simulink library "halout"  (R2021b)
settings: Solver=VariableStepAuto  StartTime=0.0  StopTime=10.0  RelTol=1e-3
undefined symbols (not defined in the file): C_TASK_5MS_S, FALSE, KHAL_CAN1TxReq_flg, KHAL_CAN2TxReq_flg, KHAL_CAN3FD3VCU1toNIDECTxReq_flg, KHAL_CAN3FD3VCU1TxReq_flg, KHAL_CAN3FD3VCU2E2E_flg, KHAL_CAN3FD3VCU2toNIDECE2E_flg, KHAL_CAN3FD3VCU2toNIDECTxReq_flg, KHAL_CAN3FD3VCU2TxReq_flg, KHAL_CAN3TxReq_flg, KHAL_CAN4FD4CE1000E2E_flg, KHAL_CAN4FD4CE1000TxReq_flg, KHAL_CAN4TxReq_flg, KHAL_CAN5TxReq_flg, KHAL_CAN7TxReq_flg, ONE_INT, TRUE, ZERO_INT
libraries: FVT_lib x258, simulink x115
(part 2 of 17)

== system halout/HAL_OUT/CAN1/GW1_C1000_1_0x18E0FF21 ==
  BSCP_outputs : Inport  OutDataTypeStr=Bus: BSCP_outputs
  BOUTP_outputs : Inport  Port=2  OutDataTypeStr=Bus: BOUTP_outputs
  SeatBeltSwitch : Subsystem
  bus_creator : BusCreator  Inputs=1  OutDataTypeStr=Bus: DT_CAN1_SG_GW1_C1000_1  NonVirtualBus=on
  bus_selector : BusSelector  OutputSignals=VOUTP_SeatBeltSwitch_enum
  GW1_C1000_1 : Outport
  wires:
  BSCP_outputs/1 -> [BSCP_outputs]
  BOUTP_outputs/1 -> [BOUTP_outputs]
  [CAN1_SeatBeltSwitch] -> bus_creator/1  "CAN1_SeatBeltSwitch"
  bus_creator/1 -> GW1_C1000_1/1
  SeatBeltSwitch/1(CAN1_SeatBeltSwitch) -> [CAN1_SeatBeltSwitch]
  bus_selector/1 -> SeatBeltSwitch/1(SeatBeltSwitch)  "<VOUTP_SeatBeltSwitch_enum>"
  [BOUTP_outputs] -> bus_selector/1

== system halout/HAL_OUT/CAN1/GW1_C100_4_0x18FDA521 ==
  BSCP_outputs : Inport  OutDataTypeStr=Bus: BSCP_outputs
  BOUTP_outputs : Inport  Port=2  OutDataTypeStr=Bus: BOUTP_outputs
  OpenStatusOfDoor1 : Subsystem
  OpenStatusOfDoor2 : Subsystem
  bus_creator : BusCreator  Inputs=2  OutDataTypeStr=Bus: DT_CAN1_SG_GW1_C100_4  NonVirtualBus=on
  bus_selector : BusSelector  OutputSignals=VOUTP_OpenStatusOfDoor1_enum
  bus_selector1 : BusSelector  OutputSignals=VOUTP_OpenStatusOfDoor2_enum
  GW1_C100_4 : Outport
  wires:
  BSCP_outputs/1 -> [BSCP_outputs]
  BOUTP_outputs/1 -> [BOUTP_outputs]
  [CAN1_OpenStatusOfDoor1] -> bus_creator/1  "CAN1_OpenStatusOfDoor1"
  [CAN1_OpenStatusOfDoor2] -> bus_creator/2  "CAN1_OpenStatusOfDoor2"
  bus_creator/1 -> GW1_C100_4/1
  OpenStatusOfDoor1/1(CAN1_OpenStatusOfDoor1) -> [CAN1_OpenStatusOfDoor1]
  OpenStatusOfDoor2/1(CAN1_OpenStatusOfDoor2) -> [CAN1_OpenStatusOfDoor2]
  bus_selector/1 -> OpenStatusOfDoor1/1(OpenStatusOfDoor1)  "<VOUTP_OpenStatusOfDoor1_enum>"
  [BOUTP_outputs] -> bus_selector/1
  bus_selector1/1 -> OpenStatusOfDoor2/1(OpenStatusOfDoor2)  "<VOUTP_OpenStatusOfDoor2_enum>"
  [BOUTP_outputs] -> bus_selector1/1

== system halout/HAL_OUT/CAN1/VCU_PDU_Demand_1_0xCF101D0 ==
  BSCP_outputs : Inport  OutDataTypeStr=Bus: BSCP_outputs
  BOUTP_outputs : Inport  Port=2  OutDataTypeStr=Bus: BOUTP_outputs
  DCDCRlyEn : Subsystem
  EACRlyEn : Subsystem
  EHPSRlyEn : Subsystem
  Ground : Ground
  VCULife1 : Subsystem
  bus_creator : BusCreator  Inputs=4  OutDataTypeStr=Bus: DT_CAN1_SG_VCU_PDU_Demand_1  NonVirtualBus=on
  bus_selector : BusSelector  OutputSignals=VOUTP_DCDCRlyDem_enum
  bus_selector1 : BusSelector  OutputSignals=VOUTP_EACRlyDem_enum
  bus_selector2 : BusSelector  OutputSignals=VOUTP_EHPSRlyDem_enum
  VCU_PDU_Demand_1 : Outport
  wires:
  BSCP_outputs/1 -> [BSCP_outputs]
  BOUTP_outputs/1 -> [BOUTP_outputs]
  [CAN1_DCDCRlyEn] -> bus_creator/1  "CAN1_DCDCRlyEn"
  [CAN1_EACRlyEn] -> bus_creator/2  "CAN1_EACRlyEn"
  [CAN1_EHPSRlyEn] -> bus_creator/3  "CAN1_EHPSRlyEn"
  [CAN1_VCULife1] -> bus_creator/4  "CAN1_VCULife1"
  bus_creator/1 -> VCU_PDU_Demand_1/1
  DCDCRlyEn/1(CAN1_DCDCRlyEn) -> [CAN1_DCDCRlyEn]
  EACRlyEn/1(CAN1_EACRlyEn) -> [CAN1_EACRlyEn]
  EHPSRlyEn/1(CAN1_EHPSRlyEn) -> [CAN1_EHPSRlyEn]
  VCULife1/1(CAN1_VCULife1) -> [CAN1_VCULife1]
  bus_selector/1 -> DCDCRlyEn/1(DCDCRlyEn)  "<VOUTP_DCDCRlyDem_enum>"
  [BOUTP_outputs] -> bus_selector/1
  bus_selector1/1 -> EACRlyEn/1(EACRlyEn)  "<VOUTP_EACRlyDem_enum>"
  [BOUTP_outputs] -> bus_selector1/1
  bus_selector2/1 -> EHPSRlyEn/1(EHPSRlyEn)  "<VOUTP_EHPSRlyDem_enum>"
  [BOUTP_outputs] -> bus_selector2/1
  Ground/1 -> VCULife1/1(VCULife1)

== system halout/HAL_OUT/CAN2/FD2_C200_1_0x18F001EF ==
  BSCP_outputs : Inport  OutDataTypeStr=Bus: BSCP_outputs
  BOUTP_outputs : Inport  Port=2  OutDataTypeStr=Bus: BOUTP_outputs
  FDCCHACACPresWarnSta : Subsystem
  FDCCHACACTempWarnSta : Subsystem
  bus_creator : BusCreator  Inputs=2  OutDataTypeStr=Bus: DT_CAN2_SG_FD2_C200_1  NonVirtualBus=on
  bus_selector : BusSelector  OutputSignals=VOUTP_CACPresWarnSta_flg
  bus_selector1 : BusSelector  OutputSignals=VOUTP_CACTempWarnSta_flg
  FD2_C200_1 : Outport
  wires:
  BSCP_outputs/1 -> [BSCP_outputs]
  BOUTP_outputs/1 -> [BOUTP_outputs]
  [CAN2_FDC_CHA_CACPresWarn_Sta] -> bus_creator/1  "CAN2_FDC_CHA_CACPresWarn_Sta"
  [CAN2_FDC_CHA_CACTempWarn_Sta] -> bus_creator/2  "CAN2_FDC_CHA_CACTempWarn_Sta"
  bus_creator/1 -> FD2_C200_1/1
  FDCCHACACPresWarnSta/1(CAN2_FDC_CHA_CACPresWarn_Sta) -> [CAN2_FDC_CHA_CACPresWarn_Sta]
  FDCCHACACTempWarnSta/1(CAN2_FDC_CHA_CACTempWarn_Sta) -> [CAN2_FDC_CHA_CACTempWarn_Sta]
  bus_selector/1 -> FDCCHACACPresWarnSta/1(FDCCHACACPresWarnSta)  "<VOUTP_CACPresWarnSta_flg>"
  [BOUTP_outputs] -> bus_selector/1
  bus_selector1/1 -> FDCCHACACTempWarnSta/1(FDCCHACACTempWarnSta)  "<VOUTP_CACTempWarnSta_flg>"
  [BOUTP_outputs] -> bus_selector1/1

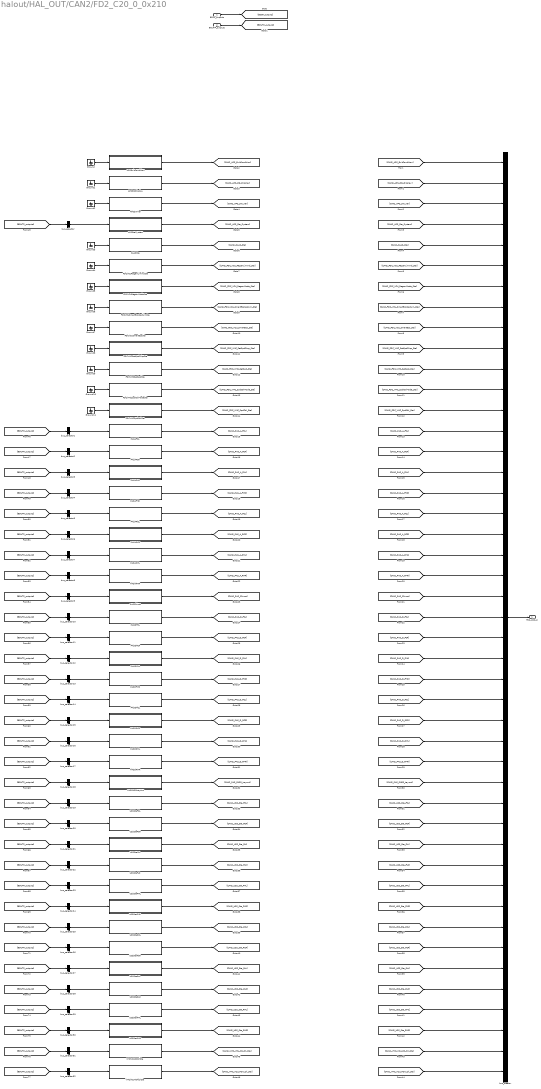
== system halout/HAL_OUT/CAN2/FD2_C20_0_0x210 ==
  BSCP_outputs : Inport  OutDataTypeStr=Bus: BSCP_outputs
  BOUTP_outputs : Inport  Port=2  OutDataTypeStr=Bus: BOUTP_outputs
  APSExitCondition : Subsystem
  APSRQDisplay : Subsystem
  APSSWVer : Subsystem
  APSStaSystem : Subsystem
  CAASSta : Subsystem
  FDCVCURegenLimIndSta : Subsystem
  FDCVCURegenModeSta : Subsystem
  FDCVCUSmartEcoSpdLimSta : Subsystem
  FDCVCUSmartEcoSta : Subsystem
  FDCVMCSetSpdDispSta : Subsystem
  FDCVMCSetSpdSta : Subsystem
  FDCVMCSpdCtrlModeSta : Subsystem
  FDCVMCSpdCtrlSta : Subsystem
  Ground{,1..11} (12 alike) : Ground
  PASAFCL : Subsystem
  PASAFCR : Subsystem
  PASAFML : Subsystem
  PASAFMR : Subsystem
  PASARCL : Subsystem
  PASARCR : Subsystem
  PASARML : Subsystem
  PASARMR : Subsystem
  PASChime : Subsystem
  PASDFCL : Subsystem
  PASDFCR : Subsystem
  PASDFML : Subsystem
  PASDFMR : Subsystem
  PASDRCL : Subsystem
  PASDRCR : Subsystem
  PASDRML : Subsystem
  PASDRMR : Subsystem
  PASSNSRLayout : Subsystem
  USSStaFCL : Subsystem
  USSStaFCR : Subsystem
  USSStaFLL : Subsystem
  USSStaFLR : Subsystem
  USSStaFML : Subsystem
  USSStaFMR : Subsystem
  USSStaRCL : Subsystem
  USSStaRCR : Subsystem
  USSStaRLL : Subsystem
  USSStaRLR : Subsystem
  USSStaRML : Subsystem
  USSStaRMR : Subsystem
  VMCVCUCCCrlSta : Subsystem
  VMCVCUMSACrlSta : Subsystem
  bus_creator : BusCreator  Inputs=45  OutDataTypeStr=Bus: DT_CAN2_SG_FD2_C20_0  NonVirtualBus=on
  bus_selector : BusSelector  OutputSignals=VOUTP_APSStaSys_enum
  bus_selector1 : BusSelector  OutputSignals=VOUTP_PASAFCL_enum
  bus_selector10 : BusSelector  OutputSignals=VOUTP_PASDFCL_cm
  bus_selector11 : BusSelector  OutputSignals=VOUTP_PASDFCR_cm
  bus_selector12 : BusSelector  OutputSignals=VOUTP_PASDFML_cm
  bus_selector13 : BusSelector  OutputSignals=VOUTP_PASDFMR_cm
  bus_selector14 : BusSelector  OutputSignals=VOUTP_PASDRCL_cm
  bus_selector15 : BusSelector  OutputSignals=VOUTP_PASDRCR_cm
  bus_selector16 : BusSelector  OutputSignals=VOUTP_PASDRML_cm
  bus_selector17 : BusSelector  OutputSignals=VOUTP_PASDRMR_cm
  bus_selector18 : BusSelector  OutputSignals=VOUTP_SNSRLayout_enum
  bus_selector19 : BusSelector  OutputSignals=VOUTP_USSStaFCL_flg
  bus_selector2 : BusSelector  OutputSignals=VOUTP_PASAFCR_enum
  bus_selector20 : BusSelector  OutputSignals=VOUTP_USSStaFCR_flg
  bus_selector21 : BusSelector  OutputSignals=VOUTP_USSStaFLL_flg
  bus_selector22 : BusSelector  OutputSignals=VOUTP_USSStaFLR_flg
  bus_selector23 : BusSelector  OutputSignals=VOUTP_USSStaFML_flg
  bus_selector24 : BusSelector  OutputSignals=VOUTP_USSStaFMR_flg
  bus_selector25 : BusSelector  OutputSignals=VOUTP_USSStaRCL_flg
  bus_selector26 : BusSelector  OutputSignals=VOUTP_USSStaRCR_flg
  bus_selector27 : BusSelector  OutputSignals=VOUTP_USSStaRLL_flg
  bus_selector28 : BusSelector  OutputSignals=VOUTP_USSStaRLR_flg
  bus_selector29 : BusSelector  OutputSignals=VOUTP_USSStaRML_flg
  bus_selector3 : BusSelector  OutputSignals=VOUTP_PASAFML_enum
  bus_selector30 : BusSelector  OutputSignals=VOUTP_USSStaRMR_flg
  bus_selector31 : BusSelector  OutputSignals=VOUTP_CCCtrlSta_enum
  bus_selector32 : BusSelector  OutputSignals=VOUTP_MSACtrlSta_enum
  bus_selector4 : BusSelector  OutputSignals=VOUTP_PASAFMR_enum
  bus_selector5 : BusSelector  OutputSignals=VOUTP_PASARCL_enum
  bus_selector6 : BusSelector  OutputSignals=VOUTP_PASARCR_enum
  bus_selector7 : BusSelector  OutputSignals=VOUTP_PASARML_enum
  bus_selector8 : BusSelector  OutputSignals=VOUTP_PASARMR_enum
  bus_selector9 : BusSelector  OutputSignals=VOUTP_Chime_enum
  FD2_C20_0 : Outport
  wires:
  BSCP_outputs/1 -> [BSCP_outputs]
  BOUTP_outputs/1 -> [BOUTP_outputs]
  [CAN2_APS_ExitCondition] -> bus_creator/1  "CAN2_APS_ExitCondition"
  [CAN2_APS_RQ_Display] -> bus_creator/2  "CAN2_APS_RQ_Display"
  [CAN2_APS_SW_Ver] -> bus_creator/3  "CAN2_APS_SW_Ver"
  [CAN2_APS_Sta_System] -> bus_creator/4  "CAN2_APS_Sta_System"
  [CAN2_CAAS_Sta] -> bus_creator/5  "CAN2_CAAS_Sta"
  [CAN2_FDC_VCU_RegenLimInd_Sta] -> bus_creator/6  "CAN2_FDC_VCU_RegenLimInd_Sta"
  [CAN2_FDC_VCU_RegenMode_Sta] -> bus_creator/7  "CAN2_FDC_VCU_RegenMode_Sta"
  [CAN2_FDC_VCU_SmartEcoSpdLim_Sta] -> bus_creator/8  "CAN2_FDC_VCU_SmartEcoSpdLim_Sta"
  [CAN2_FDC_VCU_SmartEco_Sta] -> bus_creator/9  "CAN2_FDC_VCU_SmartEco_Sta"
  [CAN2_FDC_VMC_SetSpdDisp_Sta] -> bus_creator/10  "CAN2_FDC_VMC_SetSpdDisp_Sta"
  [CAN2_FDC_VMC_SetSpd_Sta] -> bus_creator/11  "CAN2_FDC_VMC_SetSpd_Sta"
  [CAN2_FDC_VMC_SpdCtrlMode_Sta] -> bus_creator/12  "CAN2_FDC_VMC_SpdCtrlMode_Sta"
  [CAN2_FDC_VMC_SpdCtrl_Sta] -> bus_creator/13  "CAN2_FDC_VMC_SpdCtrl_Sta"
  [CAN2_PAS_A_FCL] -> bus_creator/14  "CAN2_PAS_A_FCL"
  [CAN2_PAS_A_FCR] -> bus_creator/15  "CAN2_PAS_A_FCR"
  [CAN2_PAS_A_FML] -> bus_creator/16  "CAN2_PAS_A_FML"
  [CAN2_PAS_A_FMR] -> bus_creator/17  "CAN2_PAS_A_FMR"
  [CAN2_PAS_A_RCL] -> bus_creator/18  "CAN2_PAS_A_RCL"
  [CAN2_PAS_A_RCR] -> bus_creator/19  "CAN2_PAS_A_RCR"
  [CAN2_PAS_A_RML] -> bus_creator/20  "CAN2_PAS_A_RML"
  [CAN2_PAS_A_RMR] -> bus_creator/21  "CAN2_PAS_A_RMR"
  [CAN2_PAS_Chime] -> bus_creator/22  "CAN2_PAS_Chime"
  [CAN2_PAS_D_FCL] -> bus_creator/23  "CAN2_PAS_D_FCL"
  [CAN2_PAS_D_FCR] -> bus_creator/24  "CAN2_PAS_D_FCR"
  [CAN2_PAS_D_FML] -> bus_creator/25  "CAN2_PAS_D_FML"
  [CAN2_PAS_D_FMR] -> bus_creator/26  "CAN2_PAS_D_FMR"
  [CAN2_PAS_D_RCL] -> bus_creator/27  "CAN2_PAS_D_RCL"
  [CAN2_PAS_D_RCR] -> bus_creator/28  "CAN2_PAS_D_RCR"
  [CAN2_PAS_D_RML] -> bus_creator/29  "CAN2_PAS_D_RML"
  [CAN2_PAS_D_RMR] -> bus_creator/30  "CAN2_PAS_D_RMR"
  [CAN2_PAS_SNSR_Layout] -> bus_creator/31  "CAN2_PAS_SNSR_Layout"
  [CAN2_USS_Sta_FCL] -> bus_creator/32  "CAN2_USS_Sta_FCL"
  [CAN2_USS_Sta_FCR] -> bus_creator/33  "CAN2_USS_Sta_FCR"
  [CAN2_USS_Sta_FLL] -> bus_creator/34  "CAN2_USS_Sta_FLL"
  [CAN2_USS_Sta_FLR] -> bus_creator/35  "CAN2_USS_Sta_FLR"
  [CAN2_USS_Sta_FML] -> bus_creator/36  "CAN2_USS_Sta_FML"
  [CAN2_USS_Sta_FMR] -> bus_creator/37  "CAN2_USS_Sta_FMR"
  [CAN2_USS_Sta_RCL] -> bus_creator/38  "CAN2_USS_Sta_RCL"
  [CAN2_USS_Sta_RCR] -> bus_creator/39  "CAN2_USS_Sta_RCR"
  [CAN2_USS_Sta_RLL] -> bus_creator/40  "CAN2_USS_Sta_RLL"
  [CAN2_USS_Sta_RLR] -> bus_creator/41  "CAN2_USS_Sta_RLR"
  [CAN2_USS_Sta_RML] -> bus_creator/42  "CAN2_USS_Sta_RML"
  [CAN2_USS_Sta_RMR] -> bus_creator/43  "CAN2_USS_Sta_RMR"
  [CAN2_VMC_VCU_CC_Crl_Sta] -> bus_creator/44  "CAN2_VMC_VCU_CC_Crl_Sta"
  [CAN2_VMC_VCU_MSA_Crl_Sta] -> bus_creator/45  "CAN2_VMC_VCU_MSA_Crl_Sta"
  bus_creator/1 -> FD2_C20_0/1
  APSExitCondition/1(CAN2_APS_ExitCondition) -> [CAN2_APS_ExitCondition]
  APSRQDisplay/1(CAN2_APS_RQ_Display) -> [CAN2_APS_RQ_Display]
  APSSWVer/1(CAN2_APS_SW_Ver) -> [CAN2_APS_SW_Ver]
  APSStaSystem/1(CAN2_APS_Sta_System) -> [CAN2_APS_Sta_System]
  CAASSta/1(CAN2_CAAS_Sta) -> [CAN2_CAAS_Sta]
  FDCVCURegenLimIndSta/1(CAN2_FDC_VCU_RegenLimInd_Sta) -> [CAN2_FDC_VCU_RegenLimInd_Sta]
  FDCVCURegenModeSta/1(CAN2_FDC_VCU_RegenMode_Sta) -> [CAN2_FDC_VCU_RegenMode_Sta]
  FDCVCUSmartEcoSpdLimSta/1(CAN2_FDC_VCU_SmartEcoSpdLim_Sta) -> [CAN2_FDC_VCU_SmartEcoSpdLim_Sta]
  FDCVCUSmartEcoSta/1(CAN2_FDC_VCU_SmartEco_Sta) -> [CAN2_FDC_VCU_SmartEco_Sta]
  FDCVMCSetSpdDispSta/1(CAN2_FDC_VMC_SetSpdDisp_Sta) -> [CAN2_FDC_VMC_SetSpdDisp_Sta]
  FDCVMCSetSpdSta/1(CAN2_FDC_VMC_SetSpd_Sta) -> [CAN2_FDC_VMC_SetSpd_Sta]
  FDCVMCSpdCtrlModeSta/1(CAN2_FDC_VMC_SpdCtrlMode_Sta) -> [CAN2_FDC_VMC_SpdCtrlMode_Sta]
  FDCVMCSpdCtrlSta/1(CAN2_FDC_VMC_SpdCtrl_Sta) -> [CAN2_FDC_VMC_SpdCtrl_Sta]
  PASAFCL/1(CAN2_PAS_A_FCL) -> [CAN2_PAS_A_FCL]
  PASAFCR/1(CAN2_PAS_A_FCR) -> [CAN2_PAS_A_FCR]
  PASAFML/1(CAN2_PAS_A_FML) -> [CAN2_PAS_A_FML]
  PASAFMR/1(CAN2_PAS_A_FMR) -> [CAN2_PAS_A_FMR]
  PASARCL/1(CAN2_PAS_A_RCL) -> [CAN2_PAS_A_RCL]
  PASARCR/1(CAN2_PAS_A_RCR) -> [CAN2_PAS_A_RCR]
  PASARML/1(CAN2_PAS_A_RML) -> [CAN2_PAS_A_RML]
  PASARMR/1(CAN2_PAS_A_RMR) -> [CAN2_PAS_A_RMR]
  PASChime/1(CAN2_PAS_Chime) -> [CAN2_PAS_Chime]
  PASDFCL/1(CAN2_PAS_D_FCL) -> [CAN2_PAS_D_FCL]
  PASDFCR/1(CAN2_PAS_D_FCR) -> [CAN2_PAS_D_FCR]
  PASDFML/1(CAN2_PAS_D_FML) -> [CAN2_PAS_D_FML]
  PASDFMR/1(CAN2_PAS_D_FMR) -> [CAN2_PAS_D_FMR]
  PASDRCL/1(CAN2_PAS_D_RCL) -> [CAN2_PAS_D_RCL]
  PASDRCR/1(CAN2_PAS_D_RCR) -> [CAN2_PAS_D_RCR]
  PASDRML/1(CAN2_PAS_D_RML) -> [CAN2_PAS_D_RML]
  PASDRMR/1(CAN2_PAS_D_RMR) -> [CAN2_PAS_D_RMR]
  PASSNSRLayout/1(CAN2_PAS_SNSR_Layout) -> [CAN2_PAS_SNSR_Layout]
  USSStaFCL/1(CAN2_USS_Sta_FCL) -> [CAN2_USS_Sta_FCL]
  USSStaFCR/1(CAN2_USS_Sta_FCR) -> [CAN2_USS_Sta_FCR]
  USSStaFLL/1(CAN2_USS_Sta_FLL) -> [CAN2_USS_Sta_FLL]
  USSStaFLR/1(CAN2_USS_Sta_FLR) -> [CAN2_USS_Sta_FLR]
  USSStaFML/1(CAN2_USS_Sta_FML) -> [CAN2_USS_Sta_FML]
  USSStaFMR/1(CAN2_USS_Sta_FMR) -> [CAN2_USS_Sta_FMR]
  USSStaRCL/1(CAN2_USS_Sta_RCL) -> [CAN2_USS_Sta_RCL]
  USSStaRCR/1(CAN2_USS_Sta_RCR) -> [CAN2_USS_Sta_RCR]
  USSStaRLL/1(CAN2_USS_Sta_RLL) -> [CAN2_USS_Sta_RLL]
  USSStaRLR/1(CAN2_USS_Sta_RLR) -> [CAN2_USS_Sta_RLR]
  USSStaRML/1(CAN2_USS_Sta_RML) -> [CAN2_USS_Sta_RML]
  USSStaRMR/1(CAN2_USS_Sta_RMR) -> [CAN2_USS_Sta_RMR]
  VMCVCUCCCrlSta/1(CAN2_VMC_VCU_CC_Crl_Sta) -> [CAN2_VMC_VCU_CC_Crl_Sta]
  VMCVCUMSACrlSta/1(CAN2_VMC_VCU_MSA_Crl_Sta) -> [CAN2_VMC_VCU_MSA_Crl_Sta]
  Ground/1 -> APSExitCondition/1(APSExitCondition)
  Ground1/1 -> APSRQDisplay/1(APSRQDisplay)
  Ground2/1 -> APSSWVer/1(APSSWVer)
  bus_selector/1 -> APSStaSystem/1(APSStaSystem)  "<VOUTP_APSStaSys_enum>"
  [BOUTP_outputs] -> bus_selector/1
  Ground3/1 -> CAASSta/1(CAASSta)
  Ground4/1 -> FDCVCURegenLimIndSta/1(FDCVCURegenLimIndSta)
  Ground5/1 -> FDCVCURegenModeSta/1(FDCVCURegenModeSta)
  Ground6/1 -> FDCVCUSmartEcoSpdLimSta/1(FDCVCUSmartEcoSpdLimSta)
  Ground7/1 -> FDCVCUSmartEcoSta/1(FDCVCUSmartEcoSta)
  Ground8/1 -> FDCVMCSetSpdDispSta/1(FDCVMCSetSpdDispSta)
  Ground9/1 -> FDCVMCSetSpdSta/1(FDCVMCSetSpdSta)
  Ground10/1 -> FDCVMCSpdCtrlModeSta/1(FDCVMCSpdCtrlModeSta)
  Ground11/1 -> FDCVMCSpdCtrlSta/1(FDCVMCSpdCtrlSta)
  bus_selector1/1 -> PASAFCL/1(PASAFCL)  "<VOUTP_PASAFCL_enum>"
  [BOUTP_outputs] -> bus_selector1/1
  bus_selector2/1 -> PASAFCR/1(PASAFCR)  "<VOUTP_PASAFCR_enum>"
  [BOUTP_outputs] -> bus_selector2/1
  bus_selector3/1 -> PASAFML/1(PASAFML)  "<VOUTP_PASAFML_enum>"
  [BOUTP_outputs] -> bus_selector3/1
  bus_selector4/1 -> PASAFMR/1(PASAFMR)  "<VOUTP_PASAFMR_enum>"
  [BOUTP_outputs] -> bus_selector4/1
  bus_selector5/1 -> PASARCL/1(PASARCL)  "<VOUTP_PASARCL_enum>"
  [BOUTP_outputs] -> bus_selector5/1
  bus_selector6/1 -> PASARCR/1(PASARCR)  "<VOUTP_PASARCR_enum>"
  [BOUTP_outputs] -> bus_selector6/1
  bus_selector7/1 -> PASARML/1(PASARML)  "<VOUTP_PASARML_enum>"
  [BOUTP_outputs] -> bus_selector7/1
  bus_selector8/1 -> PASARMR/1(PASARMR)  "<VOUTP_PASARMR_enum>"
  [BOUTP_outputs] -> bus_selector8/1
  bus_selector9/1 -> PASChime/1(PASChime)  "<VOUTP_Chime_enum>"
  [BOUTP_outputs] -> bus_selector9/1
  bus_selector10/1 -> PASDFCL/1(PASDFCL)  "<VOUTP_PASDFCL_cm>"
  [BOUTP_outputs] -> bus_selector10/1
  bus_selector11/1 -> PASDFCR/1(PASDFCR)  "<VOUTP_PASDFCR_cm>"
  [BOUTP_outputs] -> bus_selector11/1
  bus_selector12/1 -> PASDFML/1(PASDFML)  "<VOUTP_PASDFML_cm>"
  [BOUTP_outputs] -> bus_selector12/1
  bus_selector13/1 -> PASDFMR/1(PASDFMR)  "<VOUTP_PASDFMR_cm>"
  [BOUTP_outputs] -> bus_selector13/1
  bus_selector14/1 -> PASDRCL/1(PASDRCL)  "<VOUTP_PASDRCL_cm>"
  [BOUTP_outputs] -> bus_selector14/1
  bus_selector15/1 -> PASDRCR/1(PASDRCR)  "<VOUTP_PASDRCR_cm>"
  [BOUTP_outputs] -> bus_selector15/1
  bus_selector16/1 -> PASDRML/1(PASDRML)  "<VOUTP_PASDRML_cm>"
  [BOUTP_outputs] -> bus_selector16/1
  bus_selector17/1 -> PASDRMR/1(PASDRMR)  "<VOUTP_PASDRMR_cm>"
  [BOUTP_outputs] -> bus_selector17/1
  bus_selector18/1 -> PASSNSRLayout/1(PASSNSRLayout)  "<VOUTP_SNSRLayout_enum>"
  [BOUTP_outputs] -> bus_selector18/1
  bus_selector19/1 -> USSStaFCL/1(USSStaFCL)  "<VOUTP_USSStaFCL_flg>"
  [BOUTP_outputs] -> bus_selector19/1
  bus_selector20/1 -> USSStaFCR/1(USSStaFCR)  "<VOUTP_USSStaFCR_flg>"
  [BOUTP_outputs] -> bus_selector20/1
  bus_selector21/1 -> USSStaFLL/1(USSStaFLL)  "<VOUTP_USSStaFLL_flg>"
  [BOUTP_outputs] -> bus_selector21/1
  bus_selector22/1 -> USSStaFLR/1(USSStaFLR)  "<VOUTP_USSStaFLR_flg>"
  [BOUTP_outputs] -> bus_selector22/1
  bus_selector23/1 -> USSStaFML/1(USSStaFML)  "<VOUTP_USSStaFML_flg>"
  [BOUTP_outputs] -> bus_selector23/1
  bus_selector24/1 -> USSStaFMR/1(USSStaFMR)  "<VOUTP_USSStaFMR_flg>"
  [BOUTP_outputs] -> bus_selector24/1
  bus_selector25/1 -> USSStaRCL/1(USSStaRCL)  "<VOUTP_USSStaRCL_flg>"
  [BOUTP_outputs] -> bus_selector25/1
  bus_selector26/1 -> USSStaRCR/1(USSStaRCR)  "<VOUTP_USSStaRCR_flg>"
  [BOUTP_outputs] -> bus_selector26/1
  bus_selector27/1 -> USSStaRLL/1(USSStaRLL)  "<VOUTP_USSStaRLL_flg>"
  [BOUTP_outputs] -> bus_selector27/1
  bus_selector28/1 -> USSStaRLR/1(USSStaRLR)  "<VOUTP_USSStaRLR_flg>"
  [BOUTP_outputs] -> bus_selector28/1
  bus_selector29/1 -> USSStaRML/1(USSStaRML)  "<VOUTP_USSStaRML_flg>"
  [BOUTP_outputs] -> bus_selector29/1
  bus_selector30/1 -> USSStaRMR/1(USSStaRMR)  "<VOUTP_USSStaRMR_flg>"
  [BOUTP_outputs] -> bus_selector30/1
  bus_selector31/1 -> VMCVCUCCCrlSta/1(VMCVCUCCCrlSta)  "<VOUTP_CCCtrlSta_enum>"
  [BOUTP_outputs] -> bus_selector31/1
  bus_selector32/1 -> VMCVCUMSACrlSta/1(VMCVCUMSACrlSta)  "<VOUTP_MSACtrlSta_enum>"
  [BOUTP_outputs] -> bus_selector32/1
